simulink model "msamp1"  (Simulink 6.3)
settings: Solver=FixedStepDiscrete  StartTime=0.0  StopTime=10.0  FixedStep=0.1  RelTol=1e-3
settings Model: Creator=mshakeri  LastModifiedBy=mshakeri  ExtModeAutoUpdateStatusClock=off  StrictBusMsg=ErrorLevel1
settings OptimizationCC: InlineParams=on
settings DebuggingCC: SigSpecEnsureSampleTime=on  SignalResolutionControl=UseLocalSettings

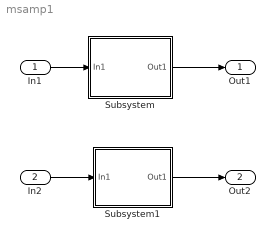
== system msamp1 ==
  In1 : Inport  Port=1  SampleTime=3  LatchInput=off  HoldInput=off
  In2 : Inport  Port=2  SampleTime=[3, 0.1]  LatchInput=off  HoldInput=off
  Subsystem : Subsystem  TreatAsAtomicUnit=on  SystemSampleTime=3
      settings: AttributesFormatString=%<SystemsampleTime>
  Subsystem1 : Subsystem  TreatAsAtomicUnit=on  SystemSampleTime=[3, 0.1]
      settings: AttributesFormatString=%<SystemSampleTime>
  Out1 : Outport
  Out2 : Outport  Port=2
  wires:
  In1/1 -> Subsystem/1(In1)
  In2/1 -> Subsystem1/1(In1)
  Subsystem/1(Out1) -> Out1/1
  Subsystem1/1(Out1) -> Out2/1

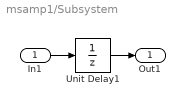
== system msamp1/Subsystem ==
  In1 : Inport  Port=1  LatchInput=off  HoldInput=off
  Unit Delay1 : UnitDelay  SampleTime=-1
  Out1 : Outport
  wires:
  In1/1 -> Unit Delay1/1
  Unit Delay1/1 -> Out1/1

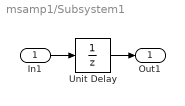
== system msamp1/Subsystem1 ==
  In1 : Inport  Port=1  LatchInput=off  HoldInput=off
  Unit Delay : UnitDelay  SampleTime=-1
  Out1 : Outport
  wires:
  In1/1 -> Unit Delay/1
  Unit Delay/1 -> Out1/1
